simulink model "LaneChangeExample"  (R2023b)
settings: Solver=VariableStepAuto  StartTime=0.0  StopTime=simStopTime  RelTol=1e-3
PostLoadFcn:
  | helperLCSetup
undefined symbols (not defined in the file): lr, m, PredictionHorizon, Ts, v_set
libraries: mpclib x1, drivingscenarioandsensors x1, autolibshared x1
CloseFcn:
  | helperLCCleanUp
settings Model: Creator=The MathWorks, Inc.  LastModifiedBy=atras
settings SolverCC: AlgebraicLoopSolver=TrustRegion
settings DebuggingCC: UnconnectedInputMsg=warning  UnconnectedOutputMsg=warning  UnconnectedLineMsg=warning
settings ModelReferenceCC: EnableRefExpFcnMdlSchedulingChecks=on
settings RTWCC: DLArmComputeVersion=19.05

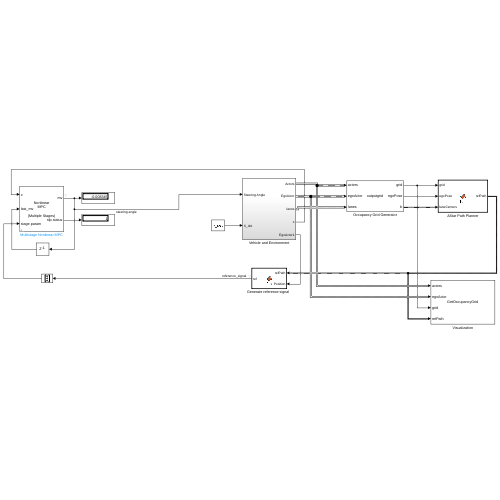
[thumbnail: Simulink's stored preview of the top-level diagram]
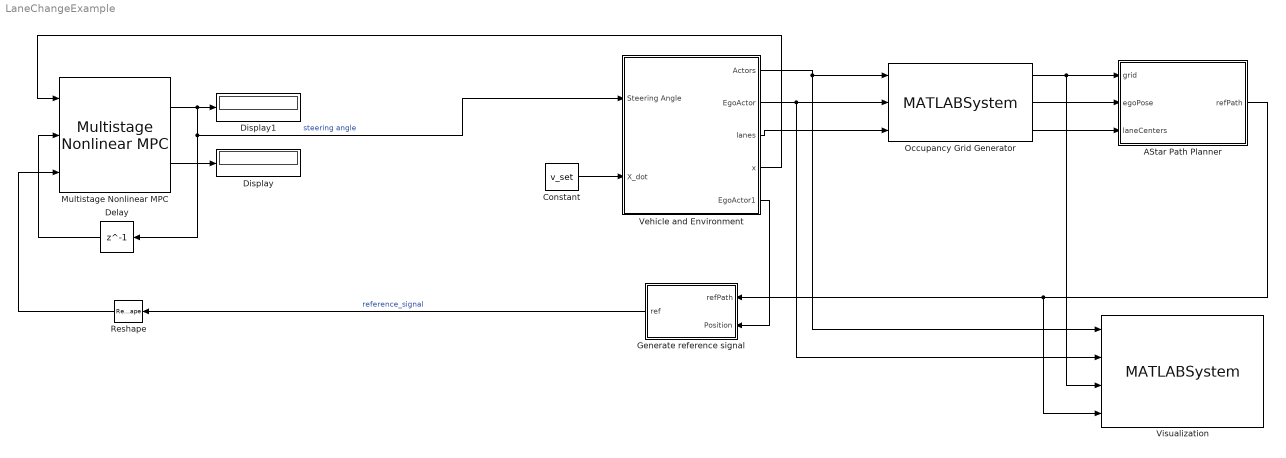
== system LaneChangeExample ==
  AStar Path Planner : MATLAB Function  TreatAsAtomicUnit=on
  Constant : Constant  Value=v_set
  Delay : Delay  DelayLength=1  InitialCondition=0
  Display : Display
  Display1 : Display
  "Generate reference signal  " : MATLAB Function  TreatAsAtomicUnit=on
  Multistage Nonlinear MPC : mpclib/Multistage Nonlinear MPC  SCDEnableBlockLinearizationSpecification=on  nlmpcobj=nlobj  UseObjectTs=on  UseMEX=off  md_enabled=off  stateparam_enabled=off  stageparam_enabled=on  cost_enabled=off  mvseq_enabled=off  stateseq_enabled=off  slack_enabled=off  status_enabled=on  mv_min=off  mv_max=off  mvrate_min=off  mvrate_max=off  state_min=off  state_max=off  terminal_state=off  nlp_initialize=off
  Occupancy Grid Generator : MATLABSystem  System=outputgrid
      mask Type: outputgrid
      mask Display:
      | disp('outputgrid');
      | port_label('input',1,'actors');
      | port_label('input',2,'egoActor');
      | port_label('input',3,'lanes');
      | port_label('output',1,'grid');
      | port_label('output',2,'egoPose');
      | port_label('output',3,'lc');
  Reshape : Reshape  OutputDimensionality=Column vector (2-D)
  Vehicle and Environment : Subsystem
  Visualization : MATLABSystem  System=GetOccupancyGrid
      mask Type: GetOccupancyGrid
      mask Display:
      | disp('GetOccupancyGrid');
      | port_label('input',1,'actors');
      | port_label('input',2,'egoActor');
      | port_label('input',3,'grid');
      | port_label('input',4,'refPath');
  wires:
  Occupancy Grid Generator/2 -> AStar Path Planner/2(egoPose)
  AStar Path Planner/1(refPath) -> Visualization/4, "Generate reference signal  "/1(refPath)
  Occupancy Grid Generator/1 -> Visualization/3, AStar Path Planner/1(grid)
  Vehicle and Environment/3(lanes) -> Occupancy Grid Generator/3
  Vehicle and Environment/1(Actors) -> Occupancy Grid Generator/1, Visualization/1
  Vehicle and Environment/2(EgoActor) -> Occupancy Grid Generator/2, Visualization/2
  Vehicle and Environment/4(x) -> Multistage Nonlinear MPC/1
  Delay/1 -> Multistage Nonlinear MPC/2
  Vehicle and Environment/5(EgoActor1) -> "Generate reference signal  "/2(Position)
  Multistage Nonlinear MPC/1 -> Delay/1, Vehicle and Environment/1(Steering Angle), Display1/1  "steering angle"
  "Generate reference signal  "/1(ref) -> Reshape/1  "reference_signal"
  Occupancy Grid Generator/3 -> AStar Path Planner/3(laneCenters)
  Multistage Nonlinear MPC/2 -> Display/1
  Reshape/1 -> Multistage Nonlinear MPC/3
  Constant/1 -> Vehicle and Environment/2(X_dot)

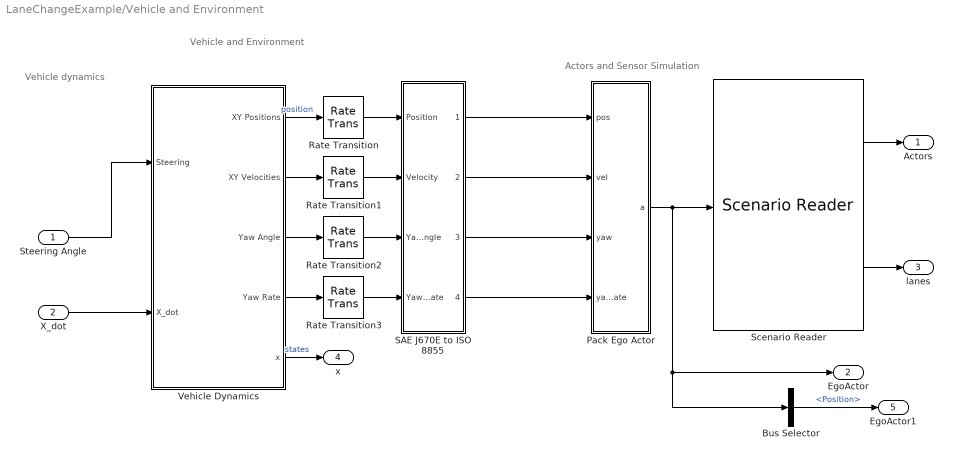
== system LaneChangeExample/Vehicle and Environment ==
  note: Vehicle dynamics
  note: Actors and Sensor Simulation
  note: Vehicle and Environment
  Steering Angle : Inport  Unit=rad
  X_dot : Inport  Port=2  Unit=m/s
  Bus Selector : BusSelector  OutputSignals=Position
  Pack Ego Actor : MATLAB Function  TreatAsAtomicUnit=on
  Rate Transition{,1..3} (4 alike) : RateTransition  OutPortSampleTime=Ts
  SAE J670E to ISO 8855 : Subsystem
  Scenario Reader : drivingscenarioandsensors/Scenario Reader  ScenarioSource=From file  ScenarioFileName=doubleLaneChangeScenario.mat  ScenarioVariableName=scenario  OutputCoordinateSystem=Vehicle coordinates  EgoVehicleSource=Input port  EgoVehicleActorID=1  OrientVehiclesOnRoad=off  OutputEgoVehiclePose=off  OutputEgoVehicleState=off  SampleTime=0.1  LaneBoundaryOutput=All lane boundaries  LaneBoundaryDistance=0:0.5:60  LaneBoundaryLocation=Center of lane markings  BusNameSource=Auto  BusName=BusActors  BusNumActorsSource=Scenario  BusNumActors=100  BusName2Source=Auto  BusName2=BusLaneBoundaries  BusNumLaneBoundariesSource=Scenario  BusNumLaneBoundaries=10  BusName3Source=Auto  BusName3=BusEgoActor  BusName4Source=Auto  BusName4=BusEgoState  ShowCoordinateLabels=on  SimulateUsing=Interpreted execution
  Vehicle Dynamics : Subsystem  VariantControl=Variant2
  Actors : Outport  VectorParamsAs1DForOutWhenUnconnected=off
  EgoActor : Outport  Port=2  VectorParamsAs1DForOutWhenUnconnected=off
  lanes : Outport  Port=3  VectorParamsAs1DForOutWhenUnconnected=off
  x : Outport  Port=4  VectorParamsAs1DForOutWhenUnconnected=off
  EgoActor1 : Outport  Port=5  VectorParamsAs1DForOutWhenUnconnected=off
  wires:
  Bus Selector/1 -> EgoActor1/1  "<Position>"
  Vehicle Dynamics/3(Yaw Angle) -> Rate Transition2/1
  Vehicle Dynamics/4(Yaw Rate) -> Rate Transition3/1
  Vehicle Dynamics/5(x) -> x/1  "states"
  Rate Transition/1 -> SAE J670E to ISO 8855/1(Position)
  Rate Transition1/1 -> SAE J670E to ISO 8855/2(Velocity)
  Rate Transition2/1 -> SAE J670E to ISO 8855/3(Yaw Angle)
  Rate Transition3/1 -> SAE J670E to ISO 8855/4(Yaw Rate)
  SAE J670E to ISO 8855/1(1) -> Pack Ego Actor/1(pos)
  SAE J670E to ISO 8855/4(4) -> Pack Ego Actor/4(yawRate)
  SAE J670E to ISO 8855/3(3) -> Pack Ego Actor/3(yaw)
  SAE J670E to ISO 8855/2(2) -> Pack Ego Actor/2(vel)
  Steering Angle/1 -> Vehicle Dynamics/1(Steering)
  Vehicle Dynamics/2(XY Velocities) -> Rate Transition1/1
  Vehicle Dynamics/1(XY Positions) -> Rate Transition/1  "position"
  Scenario Reader/1 -> Actors/1
  Scenario Reader/2 -> lanes/1
  Pack Ego Actor/1(a) -> Bus Selector/1, EgoActor/1, Scenario Reader/1
  X_dot/1 -> Vehicle Dynamics/2(X_dot)

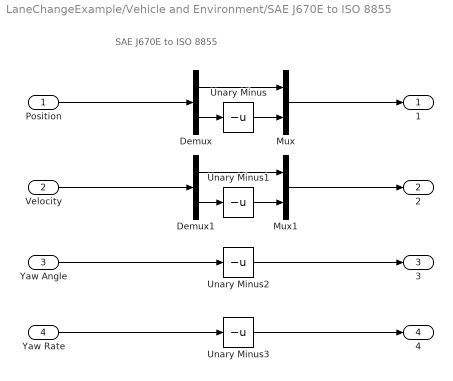
== system LaneChangeExample/Vehicle and Environment/SAE J670E to ISO 8855 ==
  note: SAE J670E to ISO 8855
  Position : Inport  Unit=m
  Velocity : Inport  Port=2  Unit=m/s
  Yaw Angle : Inport  Port=3  Unit=deg
  Yaw Rate : Inport  Port=4  Unit=deg/s
  Demux : Demux  Outputs=2
  Demux1 : Demux  Outputs=2
  Mux : Mux  Inputs=2
  Mux1 : Mux  Inputs=2
  Unary Minus{,1..3} (4 alike) : UnaryMinus
  1 : Outport  VectorParamsAs1DForOutWhenUnconnected=off
  2 : Outport  Port=2  VectorParamsAs1DForOutWhenUnconnected=off
  3 : Outport  Port=3  VectorParamsAs1DForOutWhenUnconnected=off
  4 : Outport  Port=4  VectorParamsAs1DForOutWhenUnconnected=off
  wires:
  Yaw Rate/1 -> Unary Minus3/1
  Yaw Angle/1 -> Unary Minus2/1
  Demux/1 -> Mux/1
  Demux/2 -> Unary Minus/1
  Unary Minus/1 -> Mux/2
  Unary Minus1/1 -> Mux1/2
  Demux1/2 -> Unary Minus1/1
  Demux1/1 -> Mux1/1
  Mux1/1 -> 2/1
  Mux/1 -> 1/1
  Position/1 -> Demux/1
  Velocity/1 -> Demux1/1
  Unary Minus2/1 -> 3/1
  Unary Minus3/1 -> 4/1

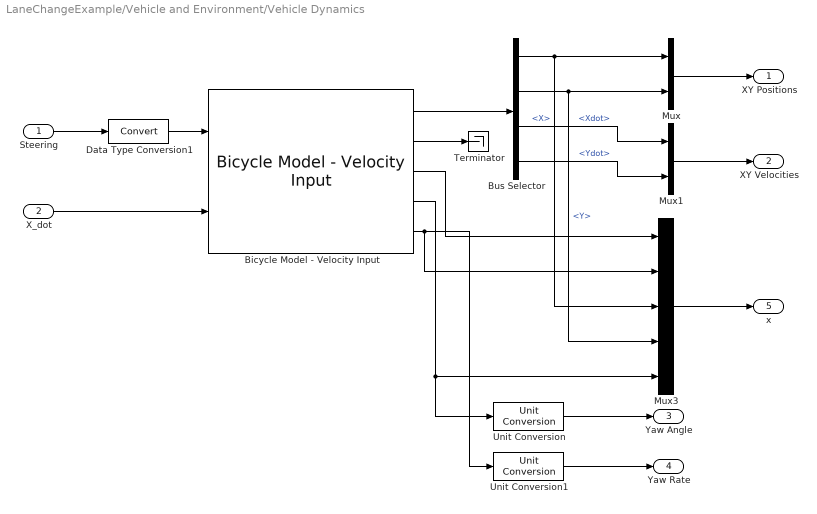
== system LaneChangeExample/Vehicle and Environment/Vehicle Dynamics ==
  Steering : Inport  Unit=rad
  X_dot : Inport  Port=2  Unit=m/s
  Bicycle Model - Velocity Input : autolibshared/Bicycle Model - Velocity Input  trackMode=Single (bicycle)  inputMode=External longitudinal velocity  frontSteerMode=on  rearSteerMode=off  windMode=off  muMode=off  extFMode=off  extMMode=off  aMode=3  NF=2  NR=2  m=m  a=lf  b=lr  h=0.35  X_o=x0_ego  xdot_o=0  CalphaMode=off  sigmaMode=on  w=[1.4,1.4]  Cy_f=Cf  Cy_r=Cr  sigma_f=.1  sigma_r=.1  alpha_f_brk=[-.1 .1]  Cy_f_data=[-9e3 9e3]  alpha_r_brk=[-.1 .1]  Cy_r_data=[-9e3 9e3]  Y_o=y0_ego  ydot_o=0  Izz=Iz  psi_o=yaw0_ego  r_o=0  Af=2  Cd=.3  Cl=.1  Cpm=.1  beta_w=[0:0.01:0.3]  Cs=[0:0.03:0.9]  Cym=[0:0.01:0.3]  Pabs=101325  Tair=273  g=9.81  mu=1  xdot_tol=.01  Fznom=5000  Fxtire_sat=1e6  Fytire_sat=1e6  longOff=0  latOff=0  vertOff=0
      settings: LibrarySourceBlock=drivingscenarioandsensors/Bicycle Model - Velocity Input
  Bus Selector : BusSelector  OutputSignals=InertFrm.FrntAxl.Disp.X,InertFrm.FrntAxl.Disp.Y,InertFrm.FrntAxl.Vel.Xdot,InertFrm.FrntAxl.Vel.Ydot
  Data Type Conversion1 : DataTypeConversion  SaturateOnIntegerOverflow=off  RndMeth=Floor
  Mux : Mux  Inputs=2
  Mux1 : Mux  Inputs=2
  Mux3 : Mux  Inputs=5
  Terminator : Terminator
  Unit Conversion : UnitConversion  OutputType=Inherit: Inherit via back propagation
  Unit Conversion1 : UnitConversion  OutputType=Inherit: Inherit via back propagation
  XY Positions : Outport  Unit=m  VectorParamsAs1DForOutWhenUnconnected=off
  XY Velocities : Outport  Port=2  Unit=m/s  VectorParamsAs1DForOutWhenUnconnected=off
  Yaw Angle : Outport  Port=3  Unit=deg  VectorParamsAs1DForOutWhenUnconnected=off
  Yaw Rate : Outport  Port=4  Unit=degree/s  VectorParamsAs1DForOutWhenUnconnected=off
  x : Outport  Port=5  VectorParamsAs1DForOutWhenUnconnected=off
  wires:
  Bicycle Model - Velocity Input/4 -> Mux3/5, Unit Conversion/1
  Bicycle Model - Velocity Input/2 -> Terminator/1
  Bicycle Model - Velocity Input/3 -> Mux3/1
  Bicycle Model - Velocity Input/1 -> Bus Selector/1
  Unit Conversion/1 -> Yaw Angle/1
  Mux3/1 -> x/1
  Unit Conversion1/1 -> Yaw Rate/1
  Data Type Conversion1/1 -> Bicycle Model - Velocity Input/1
  Bus Selector/4 -> Mux1/2  "<Ydot>"
  Mux1/1 -> XY Velocities/1
  Mux/1 -> XY Positions/1
  Bus Selector/1 -> Mux3/3, Mux/1  "<X>"
  Bus Selector/2 -> Mux3/4, Mux/2  "<Y>"
  Bus Selector/3 -> Mux1/1  "<Xdot>"
  Steering/1 -> Data Type Conversion1/1
  Bicycle Model - Velocity Input/5 -> Mux3/2, Unit Conversion1/1
  X_dot/1 -> Bicycle Model - Velocity Input/2

== matlab function LaneChangeExample/Generate reference signal   ==
  data: refPath input; ref output; Ts parameter; Position input; PredictionHorizon parameter
function ref = fcn(refPath,Ts,Position,PredictionHorizon)
% This function generates reference signal in the required format for the NMPC 

%calculating global X and Y
preview_steps = (1:PredictionHorizon)*Ts;
refPath(isnan(refPath(:)),:) =[];
if(isempty(refPath))
    % This example is designed to work for constant velocity, hence if the 
    % scenario contains slow moving  cars in all the lanes ahead of the ego car, 
    % ego car will not be able to reduce the velocity or plan a path to a
    % different lane and will error out along with the following message: 
    disp('No valid lanes available for lane change maneuver');
end
% Transfrom from Image coordinates to Ego coordinates
refPath_t = [(abs(refPath(:,1) - 800 -Position(1)/0.5)*0.5),-((refPath(:,2)- 40)*0.5)]; 
% Planner only looks ahead for 30m (2 seconds when velocity is 15m/s), if preview horizon is greater than 2 seconds
% the last value of referenc_path will be repeated
query_points = (length(refPath_t)/2)*preview_steps; % length(refPath_t/2) represent data points for 1 second
refPathc = interp1(1:length(refPath),refPath_t,round(query_points));
if(PredictionHorizon>20)
    refPathc(isnan(refPathc(:,1)),1) = refPathc(20,1);
    refPathc(isnan(refPathc(:,2)),2) = refPathc(20,2);
end
% Reference to the controller
ref = [0 refPathc(:,1)';0 -refPathc(:,2)']; % Convert ISO 8855 to SAE J670E coordinates

== matlab function LaneChangeExample/AStar Path Planner ==
  data: grid input size=[800,80]; refPath output size=[100,2]; egoPose input; laneCenters input
function refPath = fcn(grid,egoPose,laneCenters)
%#codegen

% Astar Path Planner
%
% This function plans a collision free path for the ego vehicle considering the dynamic behavior of other cars
% using Astar algorithm. This function evaluates a collision free path from the Ego Car to each of the lane 
% centers in the scenario every time step and identifies the path with the least cost and outputs (x,y) coordinates 
% of the planned path.
%
% This is a custom path planner incorporated for example purposes and may be removed or
% modified in the future.
%
% References: Astar search algorithm by Anthony Chrabieh
% https://www.mathworks.com/matlabcentral/fileexchange/64978-a-star-search-algorithm

%%
% Path Planner Initialization

% Set the starting coordinates for the planner as the current position of Ego Car
start = egoPose;

% Represent obstacles in the grid with value inf
grid(grid==1) = inf;
MAP = grid;

% Declaring variable size data for planner variables
coder.varsize('openNodes', [1000,5], [1,1]);
coder.varsize('closedNodes', [1000,5], [1,0]);
coder.varsize('path'); %, [1000,2], [1,0]);
coder.varsize('A',[1,1],[0,1]);
% Preallocate Heuristic and Movement costs
H = zeros(size(MAP,1),size(MAP,2));
G = zeros(size(MAP,1),size(MAP,2));
F = zeros(size(MAP,1),size(MAP,2));
% Variables used to compare and identify path with least cost
bestPath = [];
bestPath_cost = inf;

if(~isempty(laneCenters))
    % Remove lane center values for lanes that are not present
    laneCenters(~laneCenters) = [];
    for i=1:numel(laneCenters)
        % Planner only looks ahead for 30m (2 seconds when velocity is 15m/s),
        % hence -60 in Image Coordinates
        goal = [egoPose(1)-60, round(laneCenters(i))];
        weight = 1.5;
        % Update Heuristic vlaues of all nodes in the MAP
        for x = 1:size(MAP,1)
            for y = 1:size(MAP,2)
                if(MAP(x,y)~=inf)
                    H(x,y) = weight*norm(goal-[x,y]);
                    G(x,y) = inf;
                end
            end
        end
        
        % Initialize Moverment cost G
        G(start(1),start(2)) = 0; % s with zero
        F(start(1),start(2)) = H(start(1),start(2)); % since G is zero F= G+H = H
        % Open list and Closed list structure: [x,y,G,F,parent node]
        closedNodes = zeros(0,5);
        openNodes = [start G(start(1),start(2)) F(start(1),start(2)) 0];
        
        %%
        % Start Algorithm
        solved = false;
        while(~isempty(openNodes))
            %pause(0.001)
            % find node from open set with smallest F value
            [~,I] = min(openNodes(:,4));
            % set current node to the node with minimum function
            current = openNodes(I,:);
            % current node goal check
            if(current(1:2)==goal)
                closedNodes = [closedNodes;current];
                solved = true;
                break;
            end
            % move current node from open set to closed set
            openNodes(I,:) = [];
            closedNodes = [closedNodes;current];
            
            if(size(closedNodes,1) > 900)
                break;
            end
            
            % Expand current node
            for x = current(1)-1:current(1)+1
                for y = current(2)-1:current(2)+1
                    % node coordinate out of range check
                    if (x<1||x>size(MAP,1)||y<1||y>size(MAP,2))
                        continue
                    end
                    % node coordinate obstacle check
                    if (isinf(MAP(x,y)))
                        continue
                    end
                    % node coordinate current node check
                    if (x==current(1)&&y==current(2))
                        continue
                    end
                    % node coordinate in closed set check
                    skip = 0;
                    for j = 1:size(closedNodes,1)
                        if(x == closedNodes(j,1) && y==closedNodes(j,2))
                            skip = 1;
                            break;
                        end
                    end
                    if(skip == 1)
                        continue
                    end
                    A = zeros(1,0);
                    % node coordinate already in open set check
                    if(~isempty(openNodes))
                        for j = 1:size(openNodes,1)
                            if(x == openNodes(j,1) && y==openNodes(j,2))
                                A = j;
                                break;
                            end
                        end
                    end
                    % Update Movement cost
                    newG = G(current(1),current(2)) + 1;
                    % if not in open set, add to open set
                    if(isempty(A))
                        G(x,y) = newG;
                        newF = G(x,y) + H(x,y);
                        newNode = [x y G(x,y) newF size(closedNodes,1)];
                        openNodes = [openNodes; newNode];
                        continue
                    end
                    % check for better path
                    if (newG >= G(x,y))
                        continue
                    else
                        G(x,y) = newG;
                        newF = newG + H(x,y);
                        openNodes(A,3)= newG;
                        openNodes(A,4)= newF;
                        openNodes(A,5) = size(closedNodes,1);
                    end
                end
            end
        end
        %%
        % Evaluate planned path
        if (solved)
            j = size(closedNodes,1); %number of checked node
            path = [];
            while(j > 0)
                x = closedNodes(j,1);
                y = closedNodes(j,2);
                j = closedNodes(j,5);
                path = [x,y;path];
            end
        else
            %bestPath = repmat([egoPose(1) egoPose(2)],61,1);
            path = [];
        end
        % select path with the least cost
        if (solved && (sum(closedNodes(:,4)) < bestPath_cost))
            bestPath = path;
            bestPath_cost = sum(closedNodes(:,4));
        end
    end
else
    bestPath = [] ; 
    disp('No valid lanes available for lane change maneuver');
end
refPath = bestPath;

== matlab function LaneChangeExample/Vehicle and Environment/Pack Ego Actor ==
  data: pos input; a output Bus: BusActors1Actors size=1; vel input; yaw input; yawRate input
function a = packEgo(pos,vel,yaw,yawRate)
% Pack ego information into a single ego actor bus
%
% Imoprtant note:
% Output is a bus of type BusActorsActors. This is the same bus used by the
% Scenario Reader to output an individual actor. If you change the
% output bus name of Scenario Reader change the output bus name here
% as well by clicking on 'Edit Data' in the menu above.

a = struct(...
    'ActorID',1,...
    'Position', [pos(1) pos(2) 0], ...
    'Velocity', [vel(1) vel(2) 0], ...
    'Roll', 0, ...
    'Pitch', 0, ...
    'Yaw', yaw, ...
    'AngularVelocity', [0 0 yawRate]);
